simulink model "demowf2"  (Simulink 6.1)
settings: Solver=ode4  StartTime=0.0  StopTime=100  FixedStep=0.1  RelTol=1e-3
libraries: simulink_extras x5, simulink x3, marine_gnc x2
settings Model: LastModifiedBy=Smogeli
settings DataIOCC: SignalLoggingName=sigsOut
settings OptimizationCC: BooleanDataType=off
settings HardwareCC: TargetUnknown=on
settings GRTTargetCC: ModelReferenceCompliant=off  MatFileLogging=off

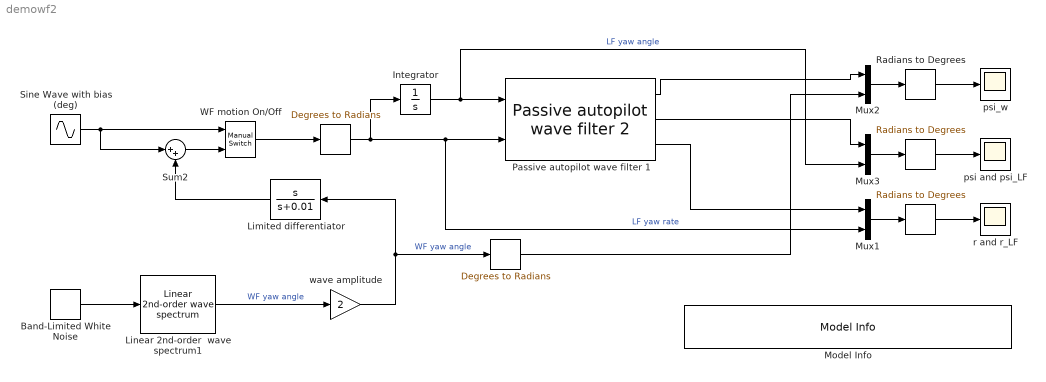
== system demowf2 ==
  " " : simulink_extras/Transformations/Radians to Degrees
  "  " : simulink_extras/Transformations/Radians to Degrees
  "   " : simulink_extras/Transformations/Degrees to Radians
  "        " : simulink_extras/Transformations/Degrees to Radians
  Band-Limited White Noise : simulink/Sources/Band-Limited White Noise  Cov=[1]  Ts=0.1  seed=[23341]
  Integrator : Integrator
  Limited differentiator : TransferFcn  Orientation=left  Numerator=[1 0]  Denominator=[1 0.01]
  Linear 2nd-order  wave spectrum1 : marine_gnc/Environment/Waves/Linear 2nd-order  wave spectrum  sigma=0.5  w_0=1.2  lambda=0.1
  Model Info : simulink/Model-Wide Utilities/Model Info  InitialBlockCM=None  BlockCM=None  Frame=on  DisplayStringWithTags=|  HorizontalTextAlignment=Left  LeftAlignmentValue=0.02  SourceBlockDiagram=demowf2  TagMaxNumber=20
      | Wave filter demo using compass and gyro measurements
      | %<Creator>Author: Thor I. Fossen
      | %<LastModificationDate>
  Mux1 : Mux  Inputs=2
  Mux2 : Mux  Inputs=2
  Mux3 : Mux  Inputs=2
  Passive autopilot wave filter 1 : marine_gnc/Navigation/Observers/Passive autopilot wave filter 2  lambda=0.1  w_o=1.2  K4=0.1  zeta_n=0.01  w_c=2  T_b=100
  "Radians to Degrees  " : simulink_extras/Transformations/Radians to Degrees
  Sine Wave with bias (deg) : Sin  Amplitude=0.5  Frequency=0.1  SampleTime=0
  Sum2 : Sum  Inputs=|++  SaturateOnIntegerOverflow=on  InputSameDT=on
  "WF motion On/Off " : simulink/Signal Routing/Manual Switch  sw=0  action=0
  psi and psi_LF : Scope
      settings: TimeRange=100  YMin=-2  YMax=12  SaveName=ScopeData2  Decimation=10
  psi_w : Scope
      settings: TimeRange=100  YMin=-3  YMax=3  Decimation=10
  r and r_LF : Scope
      settings: TimeRange=100  YMin=-3  YMax=3  SaveName=ScopeData3  Decimation=10
  wave amplitude : Gain  Gain=2  SaturateOnIntegerOverflow=on
  wires:
  Band-Limited White Noise/1 -> Linear 2nd-order  wave spectrum1/1
  Mux2/1 -> "Radians to Degrees  "/1
  "Radians to Degrees  "/1 -> psi_w/1
  " "/1 -> psi and psi_LF/1
  Mux1/1 -> "  "/1
  "  "/1 -> r and r_LF/1
  "WF motion On/Off "/1 -> "        "/1
  Linear 2nd-order  wave spectrum1/1 -> wave amplitude/1  "WF yaw angle"
  Passive autopilot wave filter 1/3 -> Mux1/1
  Integrator/1 -> Mux3/2, Passive autopilot wave filter 1/1  "LF yaw angle"
  Sine Wave with bias (deg)/1 -> "WF motion On/Off "/1, Sum2/1
  Sum2/1 -> "WF motion On/Off "/2
  "        "/1 -> Mux1/2, Passive autopilot wave filter 1/2, Integrator/1  "LF yaw rate"
  Passive autopilot wave filter 1/2 -> Mux3/1
  Mux3/1 -> " "/1
  wave amplitude/1 -> "   "/1, Limited differentiator/1  "WF yaw angle"
  Limited differentiator/1 -> Sum2/2
  Passive autopilot wave filter 1/1 -> Mux2/1
  "   "/1 -> Mux2/2
